simulink model "sche"  (R2014a)
settings: Solver=ode45  StartTime=0.0  StopTime=0.05  MaxStep=0.0001  MinStep=0.00001  RelTol=1e-3
settings Model: Creator=Valentin  LastModifiedBy=Valentin

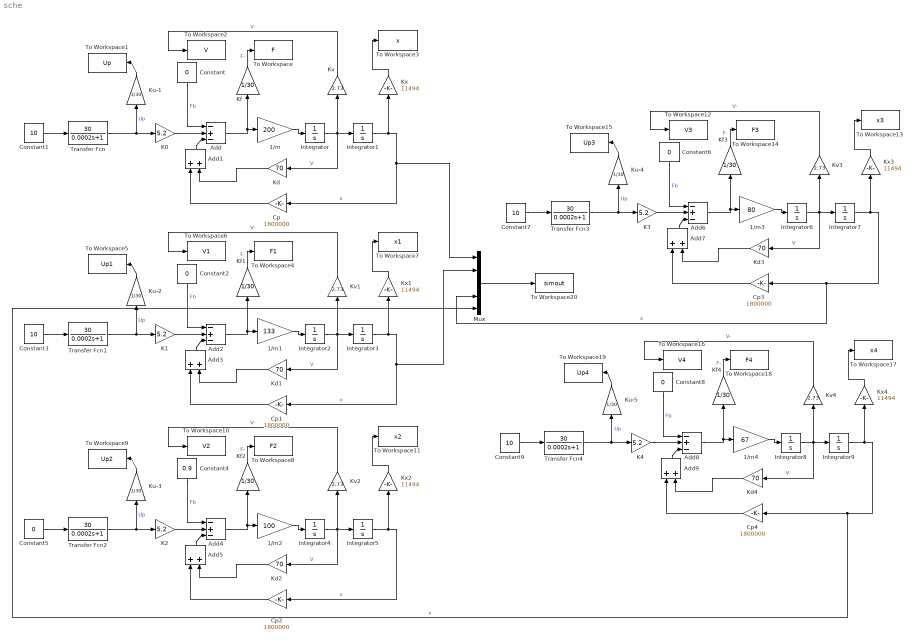
== system sche ==
  1/m : Gain  Gain=200
  1/m1 : Gain  Gain=133
  1/m2 : Gain  Gain=100
  1/m3 : Gain  Gain=80
  1/m4 : Gain  Gain=67
  Add{,2,4,6,8} (5 alike) : Sum  Inputs=-+-
  Add{1,3,5,7,9} (5 alike) : Sum
  Constant{,2,5..6,8} (5 alike) : Constant  Value=0
  Constant{1,3,7,9} (4 alike) : Constant  Value=10
  Constant4 : Constant  Value=0.9
  Cp{,1..4} (5 alike) : Gain  Gain=1800000
  Integrator{,1..9} (10 alike) : Integrator
  K{0..4} (5 alike) : Gain  Gain=5.2
  Kd{,1..4} (5 alike) : Gain  Gain=70
  Kf{,1..4} (5 alike) : Gain  Gain=1/30
  Ku-{1..5} (5 alike) : Gain  Gain=1/30
  Kv{,1..4} (5 alike) : Gain  Gain=2.73
  Kx{,1..4} (5 alike) : Gain  Gain=11494
  Mux : Mux  Inputs=5
  To Workspace : ToWorkspace  VariableName=F  SaveFormat=Timeseries  SampleTime=-1
  To Workspace1 : ToWorkspace  VariableName=Up  SaveFormat=Timeseries  SampleTime=-1
  To Workspace10 : ToWorkspace  VariableName=V2  SaveFormat=Timeseries  SampleTime=-1
  To Workspace11 : ToWorkspace  VariableName=x2  SaveFormat=Timeseries  SampleTime=-1
  To Workspace12 : ToWorkspace  VariableName=V3  SaveFormat=Timeseries  SampleTime=-1
  To Workspace13 : ToWorkspace  VariableName=x3  SaveFormat=Timeseries  SampleTime=-1
  To Workspace14 : ToWorkspace  VariableName=F3  SaveFormat=Timeseries  SampleTime=-1
  To Workspace15 : ToWorkspace  VariableName=Up3  SaveFormat=Timeseries  SampleTime=-1
  To Workspace16 : ToWorkspace  VariableName=V4  SaveFormat=Timeseries  SampleTime=-1
  To Workspace17 : ToWorkspace  VariableName=x4  SaveFormat=Timeseries  SampleTime=-1
  To Workspace18 : ToWorkspace  VariableName=F4  SaveFormat=Timeseries  SampleTime=-1
  To Workspace19 : ToWorkspace  VariableName=Up4  SaveFormat=Timeseries  SampleTime=-1
  To Workspace2 : ToWorkspace  VariableName=V  SaveFormat=Timeseries  SampleTime=-1
  To Workspace20 : ToWorkspace  VariableName=simout  SaveFormat=Timeseries  SampleTime=-1
  To Workspace3 : ToWorkspace  VariableName=x  SaveFormat=Timeseries  SampleTime=-1
  To Workspace4 : ToWorkspace  VariableName=F1  SaveFormat=Timeseries  SampleTime=-1
  To Workspace5 : ToWorkspace  VariableName=Up1  SaveFormat=Timeseries  SampleTime=-1
  To Workspace6 : ToWorkspace  VariableName=V1  SaveFormat=Timeseries  SampleTime=-1
  To Workspace7 : ToWorkspace  VariableName=x1  SaveFormat=Timeseries  SampleTime=-1
  To Workspace8 : ToWorkspace  VariableName=F2  SaveFormat=Timeseries  SampleTime=-1
  To Workspace9 : ToWorkspace  VariableName=Up2  SaveFormat=Timeseries  SampleTime=-1
  Transfer Fcn{,1..4} (5 alike) : TransferFcn  Numerator=[30]  Denominator=[0.0002 1]
  wires:
  Transfer Fcn/1 -> K0/1, Ku-1/1  "Up"
  K0/1 -> Add/2
  Cp/1 -> Add1/1
  Kd/1 -> Add1/2
  Add1/1 -> Add/3
  Add/1 -> Kf/1, 1/m/1
  1/m/1 -> Integrator/1
  Integrator/1 -> Kd/1, Kv/1, Integrator1/1  "V"
  Integrator1/1 -> Mux/1, Cp/1, Kx/1  "x"
  Ku-1/1 -> To Workspace1/1
  Constant/1 -> Add/1  "Fb"
  Kf/1 -> To Workspace/1  "F-"
  Kv/1 -> To Workspace2/1  "V-"
  Kx/1 -> To Workspace3/1
  Constant1/1 -> Transfer Fcn/1
  Transfer Fcn1/1 -> Ku-2/1, K1/1  "Up"
  K1/1 -> Add2/2
  Cp1/1 -> Add3/1
  Kd1/1 -> Add3/2
  Add3/1 -> Add2/3
  Add2/1 -> 1/m1/1, Kf1/1
  1/m1/1 -> Integrator2/1
  Integrator2/1 -> Integrator3/1, Kv1/1, Kd1/1  "V"
  Integrator3/1 -> Kx1/1, Mux/2, Cp1/1  "x"
  Ku-2/1 -> To Workspace5/1
  Constant2/1 -> Add2/1  "Fb"
  Kf1/1 -> To Workspace4/1  "F-"
  Kv1/1 -> To Workspace6/1  "V-"
  Kx1/1 -> To Workspace7/1
  Constant3/1 -> Transfer Fcn1/1
  Transfer Fcn2/1 -> K2/1, Ku-3/1  "Up"
  K2/1 -> Add4/2
  Cp2/1 -> Add5/1
  Kd2/1 -> Add5/2
  Add5/1 -> Add4/3
  Add4/1 -> Kf2/1, 1/m2/1
  1/m2/1 -> Integrator4/1
  Integrator4/1 -> Kd2/1, Kv2/1, Integrator5/1  "V"
  Integrator5/1 -> Cp2/1, Kx2/1  "x"
  Ku-3/1 -> To Workspace9/1
  Constant4/1 -> Add4/1  "Fb"
  Kf2/1 -> To Workspace8/1  "F-"
  Kv2/1 -> To Workspace10/1  "V-"
  Kx2/1 -> To Workspace11/1
  Constant5/1 -> Transfer Fcn2/1
  Transfer Fcn3/1 -> Ku-4/1, K3/1  "Up"
  K3/1 -> Add6/2
  Cp3/1 -> Add7/1
  Kd3/1 -> Add7/2
  Add7/1 -> Add6/3
  Add6/1 -> 1/m3/1, Kf3/1
  1/m3/1 -> Integrator6/1
  Integrator6/1 -> Integrator7/1, Kv3/1, Kd3/1  "V"
  Integrator7/1 -> Kx3/1, Mux/4, Cp3/1  "x"
  Ku-4/1 -> To Workspace15/1
  Constant6/1 -> Add6/1  "Fb"
  Kf3/1 -> To Workspace14/1  "F-"
  Kv3/1 -> To Workspace12/1  "V-"
  Kx3/1 -> To Workspace13/1
  Constant7/1 -> Transfer Fcn3/1
  Transfer Fcn4/1 -> K4/1, Ku-5/1  "Up"
  K4/1 -> Add8/2
  Cp4/1 -> Add9/1
  Kd4/1 -> Add9/2
  Add9/1 -> Add8/3
  Add8/1 -> Kf4/1, 1/m4/1
  1/m4/1 -> Integrator8/1
  Integrator8/1 -> Kd4/1, Kv4/1, Integrator9/1  "V"
  Integrator9/1 -> Mux/5, Cp4/1, Kx4/1  "x"
  Ku-5/1 -> To Workspace19/1
  Constant8/1 -> Add8/1  "Fb"
  Kf4/1 -> To Workspace18/1  "F-"
  Kv4/1 -> To Workspace16/1  "V-"
  Kx4/1 -> To Workspace17/1
  Constant9/1 -> Transfer Fcn4/1
  Mux/1 -> To Workspace20/1
